simulink model "recepble"  (R2020a)
settings: Solver=FixedStepAuto  StartTime=0.0  StopTime=10.0  RelTol=1e-3
undefined symbols (not defined in the file): BE, D2, F4
libraries: androiduilib x5, androidcommunicationlib x2, simulink x2
settings Model: Creator=luisi  LastModifiedBy=luisi
settings OptimizationCC: EnhancedBackFolding=on  PassReuseOutputArgsAs=Individual arguments  ZeroExternalMemoryAtStartup=off  ZeroInternalMemoryAtStartup=off  MaxStackSize=64  OptimizeBlockOrder=speed  DifferentSizesBufferReuse=on  OptimizationCustomize=off  EfficientTunableParamExpr=on
settings DebuggingCC: ParameterTunabilityLossMsg=error
settings HardwareCC: ProdBitPerPointer=32  ProdBitPerSizeT=32  ProdBitPerPtrDiffT=32  ProdLargestAtomicInteger=Long  ProdLargestAtomicFloat=Double  ProdWordSize=32  ProdHWDeviceType=ARM Compatible->ARM Cortex
settings SFSimCC: MATLABDynamicMemAlloc=off
settings RTWCC: SystemTargetFile=ert.tlc  HardwareBoard=Android Device  TemplateMakefile=ert_default_tmf  RTWVerbose=off  Toolchain=Android SDK/NDK Tools
settings CodeAppCC: ForceParamTrailComments=on  IgnoreCustomStorageClasses=off  OperatorAnnotations=on  SimulinkDataObjDesc=on  SFDataObjDesc=on  InsertBlockDesc=on

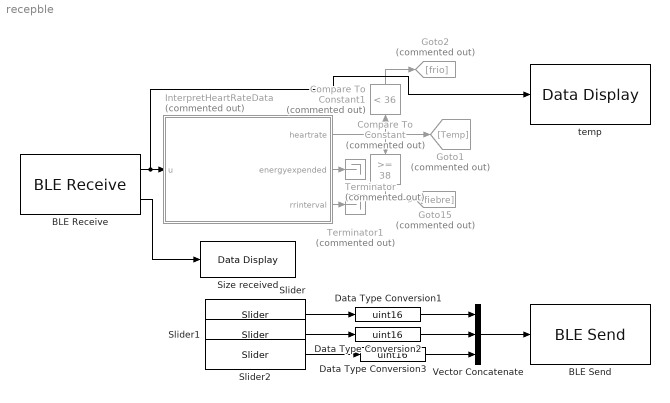
== system recepble ==
  BLE Receive : androidcommunicationlib/BLE Receive  DeviceMode=Central (Client)  BluetoothAddress=7C:F4:BE:0A:37:D2  CharUUID=0000ffe1-0000-1000-8000-00805f9b34fb  ServiceUUID=0000ffe0-0000-1000-8000-00805f9b34fb  device=RedmiJuanfe  character=0000ffe0-0000-1000-8000-00805f9b34fb\0000ffe1-0000-1000-8000-00805f9b34fb  CustomService=off  ServiceName=Heart Rate  CharacteristicName="Heart Rate  Measurement"  CustomServiceUUID=<Enter Service UUID>  CustomCharUUID=<Enter Characteristic UUID>  DataSize=7  SampleTime=0.1  charseruuid=00001801-0000-1000-8000-00805f9b34fb\00002a05-0000-1000-8000-00805f9b34fb  seruuid=00001810-0000-1000-8000-00805f9b34fb  PeripheralService=0000180d-0000-1000-8000-00805f9b34fb  PeripheralCharacteristic=00002a37-0000-1000-8000-00805f9b34fb  chruuid=00002a37-0000-1000-8000-00805f9b34fb  BLEId=recepble/BLE_Receive  Devicename=RedmiJuanfe  IsCustomService=0
      settings: SourceProductBaseCode=ANDROID
  BLE Send : androidcommunicationlib/BLE Send  DeviceMode=Central (Client)  BluetoothAddress=7C:F4:BE:0A:37:D2  CharUUID=0000fee1-0000-1000-8000-00805f9b34fb  ServiceUUID=0000ffee-0000-1000-8000-00805f9b34fb  device=RedmiJuanfe  character=0000ffee-0000-1000-8000-00805f9b34fb\0000fee1-0000-1000-8000-00805f9b34fb  CustomService=on  ServiceName=Heart Rate  CharacteristicName="Heart Rate  Measurement"  CustomServiceUUID=0000ffe0-0000-1000-8000-00805f9b34fb  CustomCharUUID=0000ffe1-0000-1000-8000-00805f9b34fb  charseruuid=00001801-0000-1000-8000-00805f9b34fb\00002a05-0000-1000-8000-00805f9b34fb  seruuid=00001810-0000-1000-8000-00805f9b34fb  chruuid=00002a37-0000-1000-8000-00805f9b34fb  PeripheralService=0000180d-0000-1000-8000-00805f9b34fb  PeripheralCharacteristic=00002a37-0000-1000-8000-00805f9b34fb  BLEId=recepble/BLE_Send  Devicename=RedmiJuanfe  IsCustomService=0  Size=-1
      settings: SourceProductBaseCode=ANDROID
  Compare To Constant : simulink/Logic and Bit Operations/Compare To Constant  Commented=on  relop=>=  const=38  OutDataTypeStr=boolean
  Compare To Constant1 : simulink/Logic and Bit Operations/Compare To Constant  Commented=on  relop=<  const=36  OutDataTypeStr=boolean
  Data Type Conversion1 : DataTypeConversion  OutDataTypeStr=uint16
  Data Type Conversion2 : DataTypeConversion  OutDataTypeStr=uint16
  Data Type Conversion3 : DataTypeConversion  OutDataTypeStr=uint16
  Goto1 : Goto  Commented=on  GotoTag=Temp
  Goto15 : Goto  Commented=on  GotoTag=fiebre
  Goto2 : Goto  Commented=on  GotoTag=frio
  InterpretHeartRateData : MATLAB Function  Commented=on  TreatAsAtomicUnit=on
  Size received : androiduilib/Data Display  DataDisplayId=recepble/Size_received  Format=Float  Precision=6  SimulateUsing=Code generation  blockPlatform=Android
      settings: SourceProductBaseCode=ANDROID
  Slider : androiduilib/Slider  Min=-5  Value=0  Max=5  Resolution=0.1  SliderId=recepble/Slider  SampleTime=0.1  BlockPlatform=Android
      settings: SourceProductBaseCode=ANDROID
  Slider1 : androiduilib/Slider  Min=-5  Value=0  Max=5  Resolution=0.1  SliderId=recepble/Slider1  SampleTime=0.1  BlockPlatform=Android
      settings: SourceProductBaseCode=ANDROID
  Slider2 : androiduilib/Slider  Min=-5  Value=0  Max=5  Resolution=0.1  SliderId=recepble/Slider2  SampleTime=0.1  BlockPlatform=Android
      settings: SourceProductBaseCode=ANDROID
  Terminator : Terminator  Commented=on
  Terminator1 : Terminator  Commented=on
  Vector Concatenate : Concatenate  NumInputs=3
  temp : androiduilib/Data Display  DataDisplayId=recepble/temp  Format=Float  Precision=6  SimulateUsing=Code generation  blockPlatform=Android
      settings: SourceProductBaseCode=ANDROID
  wires:
  InterpretHeartRateData/3(rrinterval) -> Terminator1/1
  InterpretHeartRateData/1(heartrate) -> Goto1/1, Compare To Constant1/1, Compare To Constant/1
  InterpretHeartRateData/2(energyexpended) -> Terminator/1
  Compare To Constant/1 -> Goto15/1
  BLE Receive/2 -> Size received/1
  Compare To Constant1/1 -> Goto2/1
  BLE Receive/1 -> temp/1, InterpretHeartRateData/1(u)
  Vector Concatenate/1 -> BLE Send/1
  Data Type Conversion1/1 -> Vector Concatenate/1
  Slider/1 -> Data Type Conversion1/1
  Data Type Conversion2/1 -> Vector Concatenate/2
  Slider1/1 -> Data Type Conversion2/1
  Data Type Conversion3/1 -> Vector Concatenate/3
  Slider2/1 -> Data Type Conversion3/1

== matlab function recepble/InterpretHeartRateData ==
  data: u input; heartrate output; energyexpended output; rrinterval output
function [heartrate, energyexpended, rrinterval ] = InterpretHeartRateData(u)
flag = uint8(u(1));
heartrate = uint16(0);
energyexpended=uint16(0);
rrinterval = uint16(0);
b = bitget(flag,8:-1:1);

 if b(8) == 0
     format = uint8(2);
     heartrate = uint16(u(2));
 else
     format = uint8(3);
     heartrate = typecast([u(2) u(3)], 'uint16');
 end
 
 if b(5) == 1
     energy = uint8(2);
     energyexpended = typecast([u(format +1) u(format + 2)], 'uint16');
 else
     energy = uint8(0);
     energyexpended = uint16(0);
 end
 
 if b(4) == 1
     rrinterval = typecast([u(format +energy + 1) u(format + energy + 2)],'uint16');
 else
     rrinterval = uint16(0);
 end
end
